simulink model "pueba"  (R2016b)
settings: Solver=VariableStepAuto  StartTime=0.0  StopTime=5  RelTol=1e-3
PostLoadFcn:
  | c4ModeloCompleto_var
  | set_param('pueba','AlgebraicLoopSolver','LineSearch')
values from neighbouring files (symbols this model uses):
  Beq = bm+(bl)/r^2    (= 1.5e-05)    [c4ModeloCompleto_var.m]
  Jeq = Jm+(Jl/r^2)    (= 5.65099476805e-06)    [c4ModeloCompleto_var.m]
  lambda_m = 0.01546    [c4ModeloCompleto.m]    (also in c4ModeloCompleto_var.m)
  Ld = 6.6    [c4ModeloCompleto.m]    (also in c4ModeloCompleto_var.m = 0.0066)
  Lq = 5.8    [c4ModeloCompleto.m]    (also in c4ModeloCompleto_var.m = 0.0058)
  Pp = 3    [c4ModeloCompleto.m]    (also in c4ModeloCompleto_var.m)
  r = 314.3008    [c4ModeloCompleto.m]    (also in c4ModeloCompleto_var.m)
  Rs = 1.02    [c4ModeloCompleto_var.m]
settings Model: Creator=agustin  LastModifiedBy=agustin

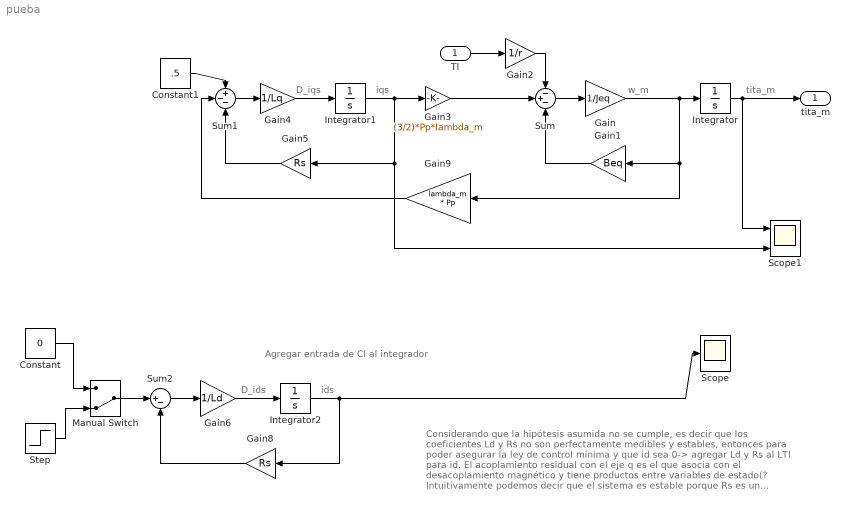
== system pueba ==
  note: Agregar entrada de CI al integrador
  note: Considerando que la hipótesis asumida no se cumple, es decir que los coeficientes Ld y Rs no son perfectamente medibles y estables, entonces para poder asegurar la ley de control mínima y que id sea 0-> agregar Ld y Rs al LTI para id.
      | El acoplamiento residual con el eje q es el que asocia con el desacoplamiento magnético y tiene productos entre variables de estado(?
      |
      | Intuitivamente podemos decir que el sistema es estable porque Rs es un término disipativo, este análisis se ve más en detalle al analizar polos.
      |
      | Se puede llegar a despreciar el acoplamiento NL porque el sistema es estable y se comporta como un filtro pasabajo con una constante de decaimiento Tau (Ld/Rs) que hace converger a la corriente a 0. El comportamiento como pasabajo se debe a que el sistema tiene un polo de primer orden
  note: ids
  note: D_ids
  note: tita_m
  note: w_m
  note: iqs
  note: D_iqs
  Tl : Inport
  Constant : Constant  Value=0
  Constant1 : Constant  Value=.5
  Gain : Gain  Gain=1/Jeq
  Gain1 : Gain  Gain=Beq
  Gain2 : Gain  Gain=1/r
  Gain3 : Gain  Gain=(3/2)*Pp*lambda_m
  Gain4 : Gain  Gain=1/Lq
  Gain5 : Gain  Gain=Rs
  Gain6 : Gain  Gain=1/Ld
  Gain8 : Gain  Gain=Rs
  Gain9 : Gain  Gain=lambda_m * Pp
  Integrator : Integrator
  Integrator1 : Integrator
  Integrator2 : Integrator
  Manual Switch : ManualSwitch  CurrentSetting=0
  Scope : Scope
  Scope1 : Scope  NumInputPorts=2
  Step : Step  Time=.1  SampleTime=0
  Sum : Sum  Inputs=-+-
  Sum1 : Sum  Inputs=+--
  Sum2 : Sum  Inputs=|+-
  tita_m : Outport
  wires:
  Gain6/1 -> Integrator2/1
  Sum2/1 -> Gain6/1
  Integrator2/1 -> Scope/1, Gain8/1
  Gain8/1 -> Sum2/2
  Constant/1 -> Manual Switch/1
  Step/1 -> Manual Switch/2
  Manual Switch/1 -> Sum2/1
  Sum/1 -> Gain/1
  Gain1/1 -> Sum/3
  Gain3/1 -> Sum/2
  Gain4/1 -> Integrator1/1
  Sum1/1 -> Gain4/1
  Integrator1/1 -> Gain3/1, Scope1/2, Gain5/1
  Gain5/1 -> Sum1/3
  Constant1/1 -> Sum1/1
  Integrator/1 -> Scope1/1, tita_m/1
  Gain/1 -> Gain9/1, Gain1/1, Integrator/1
  Gain9/1 -> Sum1/2
  Gain2/1 -> Sum/1
  Tl/1 -> Gain2/1
